simulink model "Hilly_Condition"  (R2021a)
settings: Solver=FixedStepDiscrete  StartTime=0.0  StopTime=10.0  FixedStep=0.01  RelTol=1e-3
undefined symbols (not defined in the file or in its folder): P_HillyCond_FocOn, P_HillyCond_LatDistLoLmt, P_HillyCond_LatDistUpLmt, P_HillyCond_LongiDistLoLmt, P_HillyCond_LongiDistUpLmt, P_HillyCond_SlfVehSpdLmt, P_HillyCond_SlfVehSteerAng_AClkWDi, P_HillyCond_SlfVehSteerAng_ClkWDi
settings Model: Creator=hp  LastModifiedBy=hp
settings OptimizationCC: DefaultParameterBehavior=Inlined  EnhancedBackFolding=on  PassReuseOutputArgsAs=Individual arguments  ZeroExternalMemoryAtStartup=off  ZeroInternalMemoryAtStartup=off  InitFltsAndDblsToZero=on  OptimizeBlockOrder=speed  DifferentSizesBufferReuse=on  OptimizationCustomize=off  EfficientTunableParamExpr=on
settings DebuggingCC: SignalInfNanChecking=error  CheckMatrixSingularityMsg=error  IntegerOverflowMsg=error  ParameterTunabilityLossMsg=error  UnderSpecifiedDataTypeMsg=warning  UniqueDataStoreMsg=warning  StrictBusMsg=ErrorOnBusTreatedAsVector  IntegerSaturationMsg=error
settings HardwareCC: TargetLongLongMode=on
settings SFSimCC: MATLABDynamicMemAlloc=off
settings RTWCC: SystemTargetFile=ert.tlc  TemplateMakefile=ert_default_tmf  GenerateReport=on  Toolchain=MinGW64 | gmake (64-bit Windows)  IncludeHyperlinkInReport=on  LaunchReport=on  GenerateTraceInfo=on  GenerateTraceReport=on  GenerateTraceReportSl=on  GenerateTraceReportSf=on
settings CodeAppCC: ForceParamTrailComments=on  IgnoreCustomStorageClasses=off  OperatorAnnotations=on  SimulinkDataObjDesc=on  SFDataObjDesc=on  InsertBlockDesc=on
settings ERTTargetCC: TargetLangStandard=C99 (ISO)  GenerateSampleERTMain=on  InlinedParameterPlacement=NonHierarchical  ERTCustomFileTemplate=example_file_process.tlc

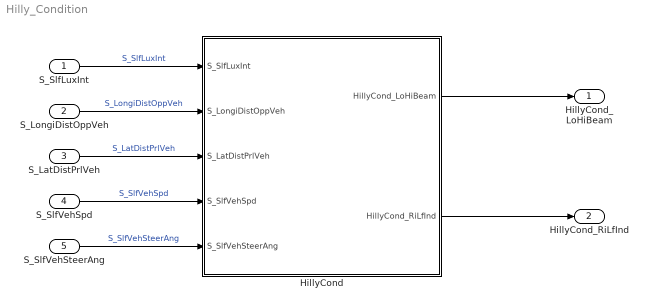
== system Hilly_Condition ==
  S_SlfLuxInt : Inport
  S_LongiDistOppVeh : Inport  Port=2
  S_LatDistPrlVeh : Inport  Port=3
  S_SlfVehSpd : Inport  Port=4
  S_SlfVehSteerAng : Inport  Port=5
  HillyCond : Subsystem  TreatAsAtomicUnit=on
  HillyCond_LoHiBeam : Outport  OutDataTypeStr=uint8
  HillyCond_RiLfInd : Outport  Port=2  OutDataTypeStr=int8
  wires:
  S_LongiDistOppVeh/1 -> HillyCond/2(S_LongiDistOppVeh)  "S_LongiDistOppVeh"
  S_LatDistPrlVeh/1 -> HillyCond/3(S_LatDistPrlVeh)  "S_LatDistPrlVeh"
  S_SlfLuxInt/1 -> HillyCond/1(S_SlfLuxInt)  "S_SlfLuxInt"
  S_SlfVehSpd/1 -> HillyCond/4(S_SlfVehSpd)  "S_SlfVehSpd"
  S_SlfVehSteerAng/1 -> HillyCond/5(S_SlfVehSteerAng)  "S_SlfVehSteerAng"
  HillyCond/1(HillyCond_LoHiBeam) -> HillyCond_LoHiBeam/1
  HillyCond/2(HillyCond_RiLfInd) -> HillyCond_RiLfInd/1

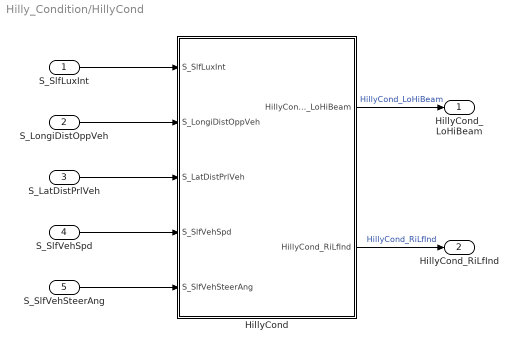
== system Hilly_Condition/HillyCond ==
  S_SlfLuxInt : Inport
  S_LongiDistOppVeh : Inport  Port=2
  S_LatDistPrlVeh : Inport  Port=3
  S_SlfVehSpd : Inport  Port=4
  S_SlfVehSteerAng : Inport  Port=5
  HillyCond : Subsystem  TreatAsAtomicUnit=on
  HillyCond_LoHiBeam : Outport
  HillyCond_RiLfInd : Outport  Port=2
  wires:
  S_SlfLuxInt/1 -> HillyCond/1(S_SlfLuxInt)
  S_LatDistPrlVeh/1 -> HillyCond/3(S_LatDistPrlVeh)
  HillyCond/1(HillyCond_LoHiBeam) -> HillyCond_LoHiBeam/1  "HillyCond_LoHiBeam"
  S_LongiDistOppVeh/1 -> HillyCond/2(S_LongiDistOppVeh)
  S_SlfVehSteerAng/1 -> HillyCond/5(S_SlfVehSteerAng)
  HillyCond/2(HillyCond_RiLfInd) -> HillyCond_RiLfInd/1  "HillyCond_RiLfInd"
  S_SlfVehSpd/1 -> HillyCond/4(S_SlfVehSpd)

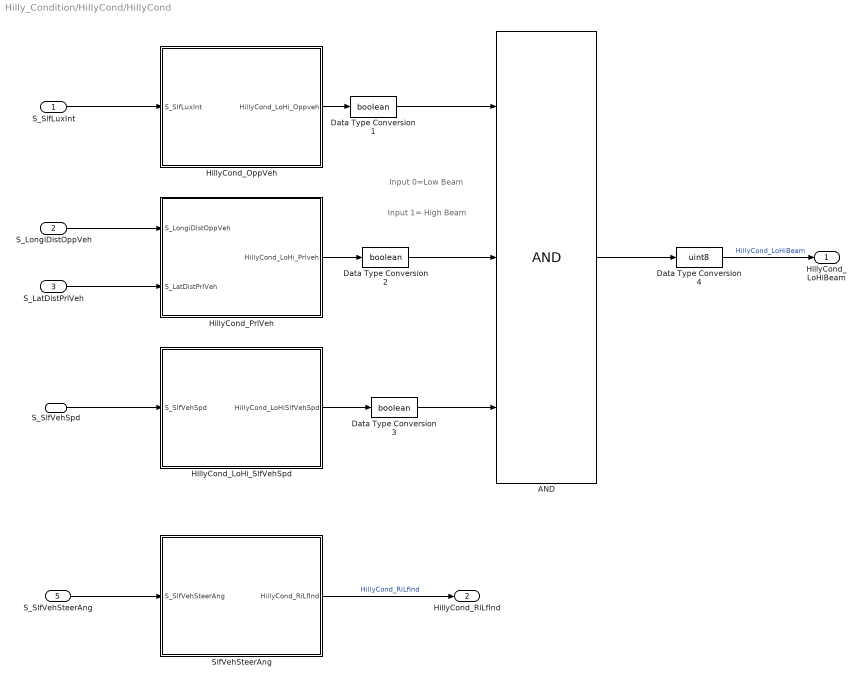
== system Hilly_Condition/HillyCond/HillyCond ==
  note: Input 0=Low Beam
  note: Input 1= High Beam
  S_SlfLuxInt : Inport
  S_LongiDistOppVeh : Inport  Port=2
  S_LatDistPrlVeh : Inport  Port=3
  S_SlfVehSpd : Inport  Port=4
  S_SlfVehSteerAng : Inport  Port=5
  AND : Logic  Inputs=3  AllPortsSameDT=off  OutDataTypeStr=boolean
  Data Type Conversion1 : DataTypeConversion  OutDataTypeStr=boolean
  Data Type Conversion2 : DataTypeConversion  OutDataTypeStr=boolean
  Data Type Conversion3 : DataTypeConversion  OutDataTypeStr=boolean
  Data Type Conversion4 : DataTypeConversion  OutDataTypeStr=uint8
  HillyCond_LoHi_SlfVehSpd : Subsystem
  HillyCond_OppVeh : Subsystem
  HillyCond_PrlVeh : Subsystem
  SlfVehSteerAng : Subsystem
  HillyCond_LoHiBeam : Outport
  HillyCond_RiLfInd : Outport  Port=2
  wires:
  S_SlfVehSteerAng/1 -> SlfVehSteerAng/1(S_SlfVehSteerAng)
  S_SlfVehSpd/1 -> HillyCond_LoHi_SlfVehSpd/1(S_SlfVehSpd)
  HillyCond_LoHi_SlfVehSpd/1(HillyCond_LoHiSlfVehSpd) -> Data Type Conversion3/1
  S_LongiDistOppVeh/1 -> HillyCond_PrlVeh/1(S_LongiDistOppVeh)
  HillyCond_OppVeh/1(HillyCond_LoHi_Oppveh) -> Data Type Conversion1/1
  S_LatDistPrlVeh/1 -> HillyCond_PrlVeh/2(S_LatDistPrlVeh)
  HillyCond_PrlVeh/1(HillyCond_LoHi_Prlveh) -> Data Type Conversion2/1
  S_SlfLuxInt/1 -> HillyCond_OppVeh/1(S_SlfLuxInt)
  AND/1 -> Data Type Conversion4/1
  SlfVehSteerAng/1(HillyCond_RiLfInd) -> HillyCond_RiLfInd/1  "HillyCond_RiLfInd"
  Data Type Conversion2/1 -> AND/2
  Data Type Conversion3/1 -> AND/3
  Data Type Conversion4/1 -> HillyCond_LoHiBeam/1  "HillyCond_LoHiBeam"
  Data Type Conversion1/1 -> AND/1

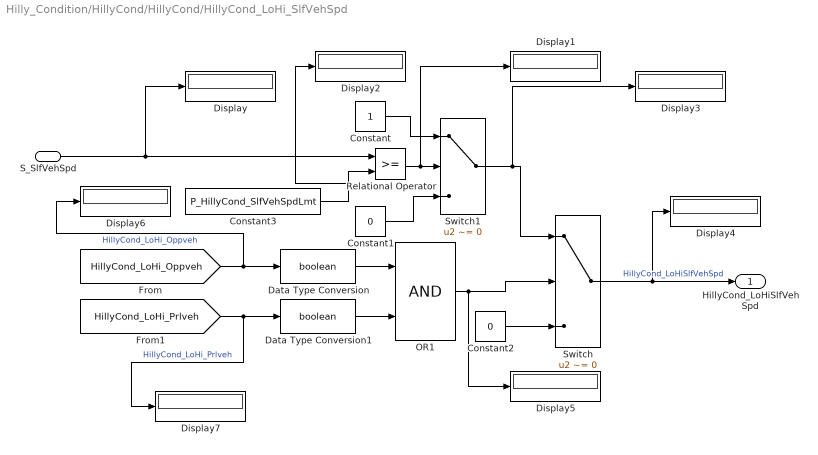
== system Hilly_Condition/HillyCond/HillyCond/HillyCond_LoHi_SlfVehSpd ==
  S_SlfVehSpd : Inport
  Constant : Constant  OutDataTypeStr=int8
  Constant1 : Constant  Value=0  OutDataTypeStr=int8
  Constant2 : Constant  Value=0  OutDataTypeStr=int8
  Constant3 : Constant  Value=P_HillyCond_SlfVehSpdLmt
  Data Type Conversion : DataTypeConversion  OutDataTypeStr=boolean
  Data Type Conversion1 : DataTypeConversion  OutDataTypeStr=boolean
  Display{,1..7} (8 alike) : Display
  OR1 : Logic  AllPortsSameDT=off  OutDataTypeStr=boolean
  Relational Operator : RelationalOperator  OutDataTypeStr=boolean  RndMeth=Simplest
  Switch : Switch  Criteria=u2 ~= 0  OutDataTypeStr=Inherit: Inherit via back propagation
  Switch1 : Switch  Criteria=u2 ~= 0
  HillyCond_LoHiSlfVehSpd : Outport  OutDataTypeStr=int8
  wires:
  OR1/1 -> Display5/1, Switch/2
  [HillyCond_LoHi_Prlveh] -> Display7/1, Data Type Conversion1/1  "HillyCond_LoHi_Prlveh"
  S_SlfVehSpd/1 -> Display/1, Relational Operator/1
  Switch/1 -> Display4/1, HillyCond_LoHiSlfVehSpd/1  "HillyCond_LoHiSlfVehSpd"
  Switch1/1 -> Display3/1, Switch/1
  Constant2/1 -> Switch/3
  Constant/1 -> Switch1/1
  Relational Operator/1 -> Display1/1, Switch1/2
  Constant1/1 -> Switch1/3
  [HillyCond_LoHi_Oppveh] -> Display6/1, Data Type Conversion/1  "HillyCond_LoHi_Oppveh"
  Constant3/1 -> Display2/1, Relational Operator/2
  Data Type Conversion/1 -> OR1/1
  Data Type Conversion1/1 -> OR1/2

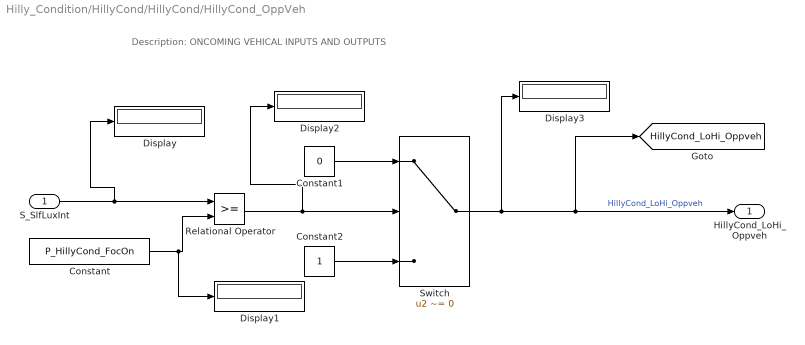
== system Hilly_Condition/HillyCond/HillyCond/HillyCond_OppVeh ==
  note: Description: ONCOMING VEHICAL INPUTS AND OUTPUTS
  S_SlfLuxInt : Inport
  Constant : Constant  Value=P_HillyCond_FocOn
  Constant1 : Constant  Value=0  OutDataTypeStr=int8
  Constant2 : Constant  OutDataTypeStr=int8
  Display{,1..3} (4 alike) : Display
  Relational Operator : RelationalOperator  OutDataTypeStr=boolean  RndMeth=Simplest
  Switch : Switch  Criteria=u2 ~= 0
  HillyCond_LoHi_Oppveh : Outport  OutDataTypeStr=int8
  tag scope: HillyCond_LoHi_Oppveh=global
  wires:
  Constant2/1 -> Switch/3
  Constant1/1 -> Switch/1
  Switch/1 -> Display3/1, HillyCond_LoHi_Oppveh/1, [HillyCond_LoHi_Oppveh]  "HillyCond_LoHi_Oppveh"
  S_SlfLuxInt/1 -> Display/1, Relational Operator/1
  Relational Operator/1 -> Display2/1, Switch/2
  Constant/1 -> Display1/1, Relational Operator/2

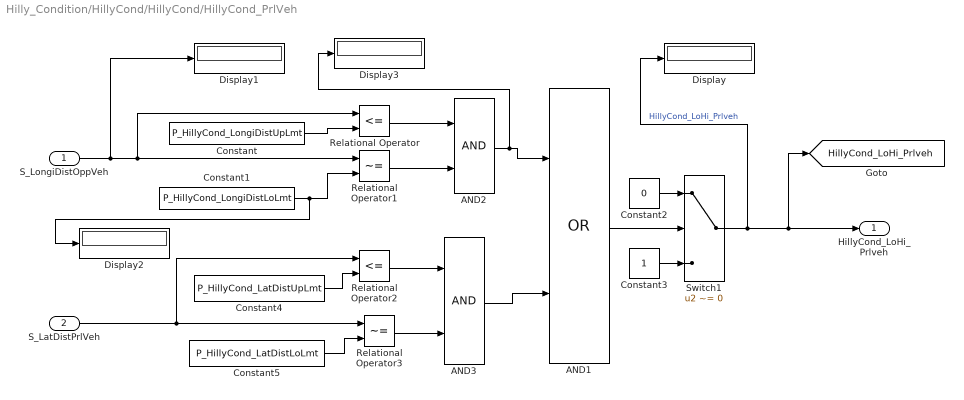
== system Hilly_Condition/HillyCond/HillyCond/HillyCond_PrlVeh ==
  S_LongiDistOppVeh : Inport
  S_LatDistPrlVeh : Inport  Port=2
  AND1 : Logic  Operator=OR  AllPortsSameDT=off  OutDataTypeStr=boolean
  AND2 : Logic  AllPortsSameDT=off  OutDataTypeStr=boolean
  AND3 : Logic  AllPortsSameDT=off  OutDataTypeStr=boolean
  Constant : Constant  Value=P_HillyCond_LongiDistUpLmt
  Constant1 : Constant  Value=P_HillyCond_LongiDistLoLmt
  Constant2 : Constant  Value=0  OutDataTypeStr=int8
  Constant3 : Constant  OutDataTypeStr=int8
  Constant4 : Constant  Value=P_HillyCond_LatDistUpLmt
  Constant5 : Constant  Value=P_HillyCond_LatDistLoLmt
  Display{,1..3} (4 alike) : Display
  Relational Operator : RelationalOperator  Operator=<=  OutDataTypeStr=boolean  RndMeth=Simplest
  Relational Operator1 : RelationalOperator  Operator=~=  OutDataTypeStr=boolean  RndMeth=Simplest
  Relational Operator2 : RelationalOperator  Operator=<=  OutDataTypeStr=boolean  RndMeth=Simplest
  Relational Operator3 : RelationalOperator  Operator=~=  OutDataTypeStr=boolean  RndMeth=Simplest
  Switch1 : Switch  Criteria=u2 ~= 0
  HillyCond_LoHi_Prlveh : Outport  OutDataTypeStr=int8
  tag scope: HillyCond_LoHi_Prlveh=global
  wires:
  Constant3/1 -> Switch1/3
  Constant2/1 -> Switch1/1
  AND2/1 -> Display3/1, AND1/1
  Switch1/1 -> Display/1, HillyCond_LoHi_Prlveh/1, [HillyCond_LoHi_Prlveh]  "HillyCond_LoHi_Prlveh"
  AND1/1 -> Switch1/2
  S_LatDistPrlVeh/1 -> Relational Operator3/1, Relational Operator2/1
  S_LongiDistOppVeh/1 -> Display1/1, Relational Operator/1, Relational Operator1/1
  Constant/1 -> Relational Operator/2
  Relational Operator/1 -> AND2/1
  Constant1/1 -> Display2/1, Relational Operator1/2
  Relational Operator1/1 -> AND2/2
  Constant4/1 -> Relational Operator2/2
  Relational Operator2/1 -> AND3/1
  AND3/1 -> AND1/2
  Constant5/1 -> Relational Operator3/2
  Relational Operator3/1 -> AND3/2

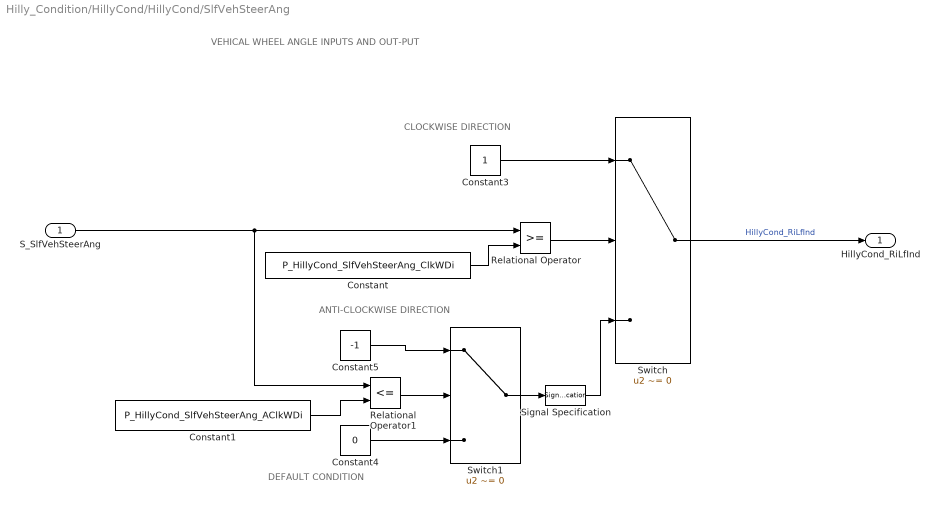
== system Hilly_Condition/HillyCond/HillyCond/SlfVehSteerAng ==
  note: ANTI-CLOCKWISE DIRECTION
  note: VEHICAL WHEEL ANGLE INPUTS AND OUT-PUT
  note: CLOCKWISE DIRECTION
  note: DEFAULT CONDITION
  S_SlfVehSteerAng : Inport
  Constant : Constant  Value=P_HillyCond_SlfVehSteerAng_ClkWDi
  Constant1 : Constant  Value=P_HillyCond_SlfVehSteerAng_AClkWDi
  Constant3 : Constant  OutDataTypeStr=int8
  Constant4 : Constant  Value=0  OutDataTypeStr=int8
  Constant5 : Constant  Value=-1  OutDataTypeStr=int8
  Relational Operator : RelationalOperator  OutDataTypeStr=boolean  RndMeth=Simplest
  Relational Operator1 : RelationalOperator  Operator=<=  OutDataTypeStr=boolean  RndMeth=Simplest
  Signal Specification : SignalSpecification  OutDataTypeStr=int8
      settings: LockScale=on
  Switch : Switch  Criteria=u2 ~= 0  OutDataTypeStr=Inherit: Inherit via back propagation
  Switch1 : Switch  Criteria=u2 ~= 0  OutDataTypeStr=Inherit: Inherit via back propagation
  HillyCond_RiLfInd : Outport  OutDataTypeStr=int8
  wires:
  S_SlfVehSteerAng/1 -> Relational Operator1/1, Relational Operator/1
  Constant3/1 -> Switch/1
  Constant5/1 -> Switch1/1
  Constant4/1 -> Switch1/3
  Switch/1 -> HillyCond_RiLfInd/1  "HillyCond_RiLfInd"
  Constant/1 -> Relational Operator/2
  Relational Operator/1 -> Switch/2
  Constant1/1 -> Relational Operator1/2
  Relational Operator1/1 -> Switch1/2
  Switch1/1 -> Signal Specification/1
  Signal Specification/1 -> Switch/3
